simulink model "mag"  (R2020a)
settings: Solver=VariableStepAuto  StartTime=0.0  StopTime=10.0  RelTol=1e-3
undefined symbols (not defined in the file or in its folder): magneticConstants
settings Model: Creator=tomis  LastModifiedBy=tomis

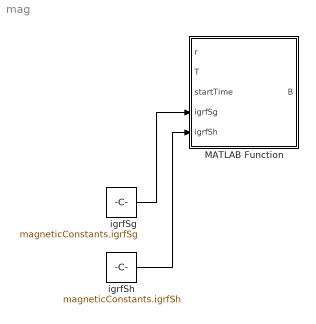
== system mag ==
  MATLAB Function : MATLAB Function  TreatAsAtomicUnit=on
  igrfSg : Constant  Value=magneticConstants.igrfSg
  igrfSh : Constant  Value=magneticConstants.igrfSh
  wires:
  igrfSg/1 -> MATLAB Function/4(igrfSg)
  igrfSh/1 -> MATLAB Function/5(igrfSh)

== matlab function mag/MATLAB Function ==
  data: r input; B output; T input; startTime input; igrfSg input; igrfSh input
function B = fcn(r, T, startTime, igrfSg, igrfSh)

days = startTime + T/86400;

[rNorm, lat, lon] = carToGCS(r, T);
[Br,Bt,Bp] = magnet(rNorm,lat,lon,days,igrfSg,igrfSh);
[Bx,By,Bz] = msph2inert(Br,Bt,Bp,LST,lat);
B = [Bx; By; Bz];
end
